simulink model "comproject"  (R2024a)
settings: Solver=VariableStepAuto  StartTime=0.0  StopTime=0.01  MaxStep=0.001  RelTol=1e-3
undefined symbols (not defined in the file): fdesignblkfcn, gcbh
libraries: simulink x4, dspfdesign x2
settings Model: Creator=Sazzad Hossen  LastModifiedBy=Sazzad Hossen

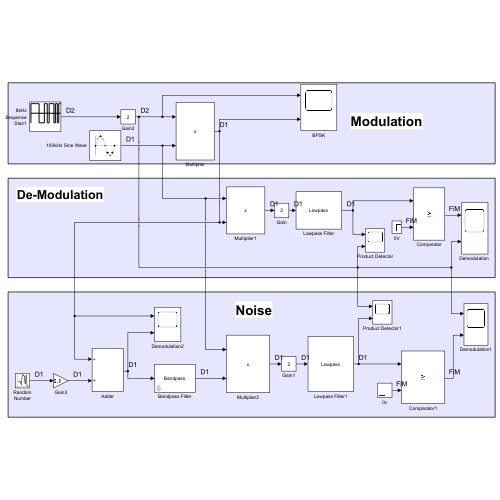
[thumbnail: Simulink's stored preview of the top-level diagram]
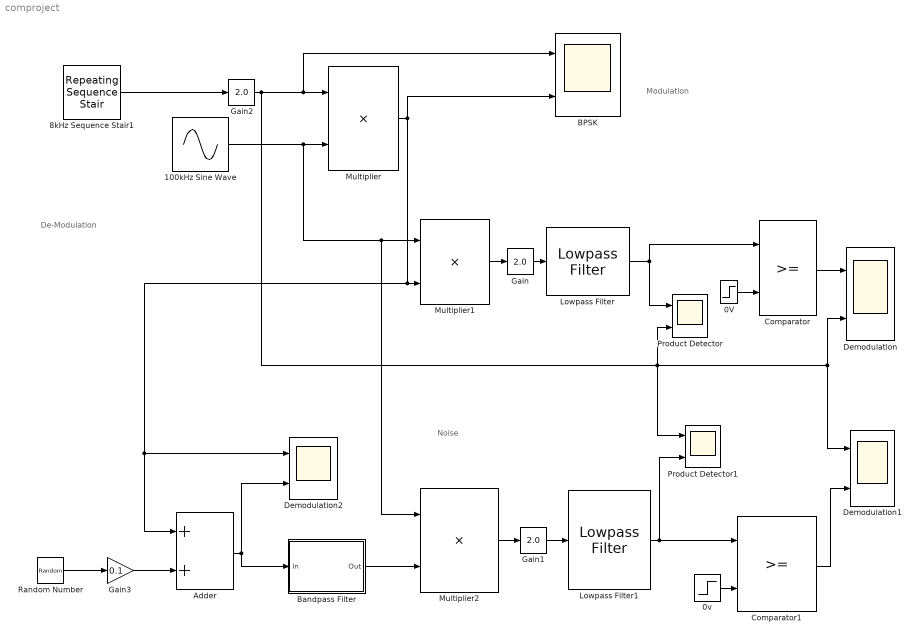
== system comproject ==
  note: Modulation
  note: De-Modulation
  note: Noise
  0V : Step  Time=0  After=0  SampleTime=0
  0v : Step  Time=0  After=0  SampleTime=0
  100kHz Sine Wave : Sin  SineType=Sample based  SampleTime=1e-6
  8kHz Sequence Stair1 : simulink/Sources/Repeating Sequence Stair  OutValues=[1 1 1 1 1 -1 -1 -1 1 1 -1 1 1 1 -1 +1 -1 +1].'  tsamp=1/8000  OutMin=[]  OutMax=[]  OutDataTypeStr=double  OutputDataTypeScalingMode=double  OutDataType=fixdt(0,8)  ConRadixGroup=Best Precision: Vector-wise  OutScaling=2^-12
  Adder : Sum
  BPSK : Scope  NumInputPorts=2
  Bandpass Filter : Subsystem  DialogController=fdesignblkfcn  InitFcn=fdesignblkfcn(gcbh, {'InitFcn'});  mask(Bandpass Filter){}
      mask help: dsp:DSPFilterDesignBlockDialog:BandpassFdesign_MaskDesc
      settings: CopyFcn=fdesignblkfcn(gcbh, {'CopyFcn'});
      mask Help: helpview(mapfilelocation('dsp'), 'dspbandpassfilter');
      mask Display: disp('Bandpass');
  Comparator : RelationalOperator  OutDataTypeStr=boolean  RndMeth=Simplest  InputSameDT=off
  Comparator1 : RelationalOperator  OutDataTypeStr=boolean  RndMeth=Simplest  InputSameDT=off
  "Demodulation " : Scope  NumInputPorts=2
  Demodulation1 : Scope  NumInputPorts=2
  Demodulation2 : Scope  NumInputPorts=2
  Gain : simulink/Math Operations/Slider Gain  gain=2.0  low=0  high=2
  Gain1 : simulink/Math Operations/Slider Gain  gain=2.0  low=0  high=2
  Gain2 : simulink/Math Operations/Slider Gain  gain=2.0  low=0  high=2
  Gain3 : Gain  Gain=0.1
  Lowpass Filter : dspfdesign/Lowpass Filter  FilterType=IIR  DesignForMinimumOrder=on  FilterOrder=50  PassbandFrequency=6e3  StopbandFrequency=10e3  PassbandRipple=3  StopbandAttenuation=20  SampleRateMode=Specify on dialog  SampleRate=1000000  SimulateUsing=Interpreted execution  roundingMode=Floor  coeffsDataTypeStr=fixdt(1,16)
  Lowpass Filter1 : dspfdesign/Lowpass Filter  FilterType=IIR  DesignForMinimumOrder=on  FilterOrder=50  PassbandFrequency=6e3  StopbandFrequency=10e3  PassbandRipple=3  StopbandAttenuation=80  SampleRateMode=Specify on dialog  SampleRate=1000000  SimulateUsing=Interpreted execution  roundingMode=Floor  coeffsDataTypeStr=fixdt(1,16)
  Multiplier : Product
  Multiplier1 : Product
  Multiplier2 : Product
  Product Detector : Scope  NumInputPorts=2
  Product Detector1 : Scope  NumInputPorts=2
  Random Number : RandomNumber  SampleTime=1e-6
  wires:
  100kHz Sine Wave/1 -> Multiplier1/1, Multiplier2/1, Multiplier/2
  Multiplier/1 -> Demodulation2/1, Adder/1, Multiplier1/2, BPSK/2
  Multiplier1/1 -> Gain/1
  Gain/1 -> Lowpass Filter/1
  Lowpass Filter/1 -> Comparator/1, Product Detector/1
  Comparator/1 -> "Demodulation "/1
  Adder/1 -> Bandpass Filter/1(In), Demodulation2/2
  Gain1/1 -> Lowpass Filter1/1
  Multiplier2/1 -> Gain1/1
  Gain3/1 -> Adder/2
  Bandpass Filter/1(Out) -> Multiplier2/2
  Lowpass Filter1/1 -> Product Detector1/2, Comparator1/1
  0v/1 -> Comparator1/2
  Comparator1/1 -> Demodulation1/2
  0V/1 -> Comparator/2
  Gain2/1 -> BPSK/1, Multiplier/1, Product Detector/2, "Demodulation "/2, Demodulation1/1, Product Detector1/1
  8kHz Sequence Stair1/1 -> Gain2/1
  Random Number/1 -> Gain3/1

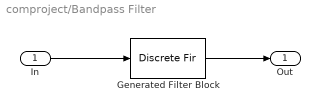
== system comproject/Bandpass Filter ==
  In : Inport
  Generated Filter Block : DiscreteFir  Tag=BlockMethodSubSystem  Coefficients=[-0.00089884629803854883 0.00164204827488956132 0.00313280207602157192 -0.00406942058599144788 -0.00636638984575240915 0.00748358323475895211 0.00982265765831517694 -0.010181761336883012 -0.0112842317755903285 0.00968051905136860236 0.00792119831891151954 -0.00312033955811022098 0.00285217817894855424 -0.0115282222059956488 -0.0220982481350457879 0.0342641500023354931 0.0483679667777207403 -0.0623695016169409436 -0.0775063823718388778 0.0906949609287212438 0.103527564982536457 -0.112978430596438598 -0.120351411155716112 0.12378776347897899 0.12378776347897899 -0.120351411155716112 -0.112978430596438598 0.103527564982536457 0.0906949609287212438 -0.0775063823718388778 -0.0623695016169409436 0.0483679667777207403 0.0342641500023354931 -0.0220982481350457879 -0.0115282222059956488 0.00285217817894855424 -0.00312033955811022098 0.00792119831891151954 0.00968051905136860236 -0.0112842317755903285 -0.010181761336883012 0.00982265765831517694 0.00748358323475895211 -0.00636638984575240915 -0.00406942058599144788 0.00313280207602157192 0.00164204827488956132 -0.00089884629803854883]  InputProcessing=Columns as channels (frame based)
  Out : Outport  VectorParamsAs1DForOutWhenUnconnected=off
  wires:
  In/1 -> Generated Filter Block/1
  Generated Filter Block/1 -> Out/1
